simulink subsystem "neg_yarn_feeder_model"  (R2023b)
settings: Solver=VariableStepAuto  StartTime=0.0  StopTime=10.0  RelTol=1e-3
libraries: cstblocks x1
settings Model: Creator=Previ  LastModifiedBy=Previ

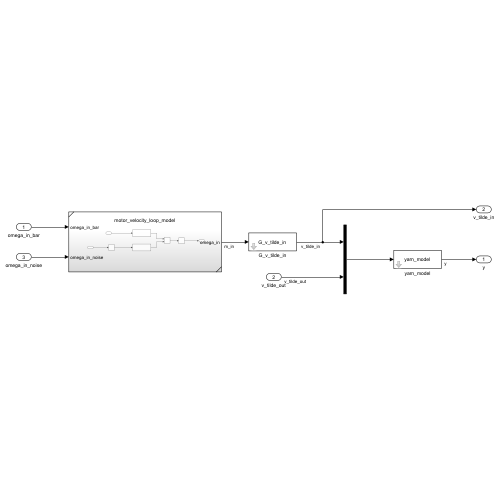
[thumbnail: Simulink's stored preview of the top-level diagram]
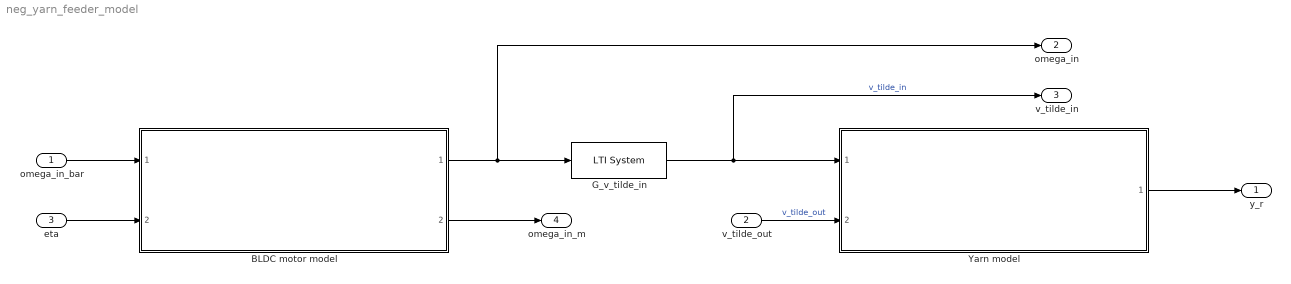
== system neg_yarn_feeder_model ==
  omega_in_bar : Inport  PortDimensions=[1, 1]
  v_tilde_out : Inport  Port=2  PortDimensions=[1, 1]
  eta : Inport  Port=3  PortDimensions=[1, 1]
  BLDC motor model : Subsystem  ReferencedSubsystem=motor_velocity_loop_model
  G_v_tilde_in : cstblocks/LTI System  sys=G_v_tilde_in  IC=[]  PadeOrder=0
  Yarn model : Subsystem  ReferencedSubsystem=yarn_model
  y_r : Outport  PortDimensions=[1, 1]
  omega_in : Outport  Port=2  PortDimensions=[1, 1]
  v_tilde_in : Outport  Port=3  PortDimensions=[1, 1]
  omega_in_m : Outport  Port=4  PortDimensions=[1, 1]
  wires:
  G_v_tilde_in/1 -> Yarn model/1, v_tilde_in/1  "v_tilde_in"
  omega_in_bar/1 -> BLDC motor model/1
  eta/1 -> BLDC motor model/2
  BLDC motor model/1 -> G_v_tilde_in/1, omega_in/1
  v_tilde_out/1 -> Yarn model/2  "v_tilde_out"
  Yarn model/1 -> y_r/1
  BLDC motor model/2 -> omega_in_m/1
